simulink subsystem "QuaternionUpdate"  (R2021a)
settings: Solver=VariableStepAuto  StartTime=0.0  StopTime=10.0  RelTol=1e-3
libraries: aerolibutil x1, sharedutil x1, attitude_library x1
settings Model: Creator=Laura  LastModifiedBy=Laura

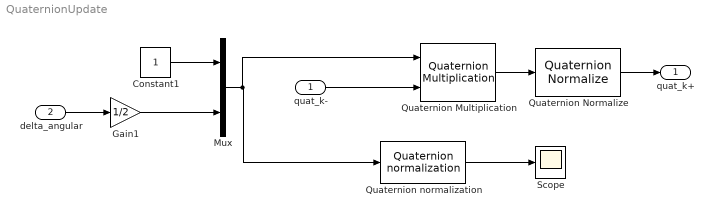
== system QuaternionUpdate ==
  quat_k- : Inport
  delta_angular : Inport  Port=2
  Constant1 : Constant
  Gain1 : Gain  Gain=1/2
  Mux : Mux  Inputs=2
  Quaternion Multiplication : aerolibutil/Quaternion Multiplication
  Quaternion Normalize : sharedutil/Quaternion Normalize  aMode=aMode
      settings: SourceProductBaseCode=AE,PW,DR,MT,UV,VE
  Quaternion normalization : attitude_library/Quaternion normalization  SystemSampleTime=-1  VariantActivationTime=update diagram  Latency=0  AutoFrameSizeCalculation=off
      settings: SourceProductName=Attitude library
  Scope : Scope
  quat_k+ : Outport
  wires:
  Quaternion Normalize/1 -> quat_k+/1
  Quaternion Multiplication/1 -> Quaternion Normalize/1
  Quaternion normalization/1 -> Scope/1
  Mux/1 -> Quaternion normalization/1, Quaternion Multiplication/1
  Gain1/1 -> Mux/2
  Constant1/1 -> Mux/1
  delta_angular/1 -> Gain1/1
  quat_k-/1 -> Quaternion Multiplication/2
